simulink subsystem "Get_Lanes_and_Return_Map"  (R2022b)
settings: Solver=VariableStepAuto  StartTime=0.0  StopTime=10.0  RelTol=1e-3
settings Model: Creator=User  LastModifiedBy=User

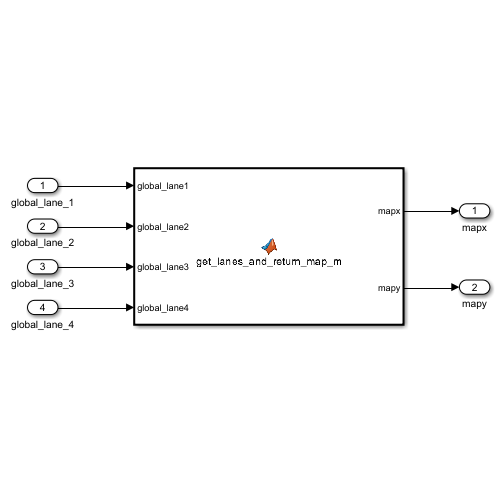
[thumbnail: Simulink's stored preview of the top-level diagram]
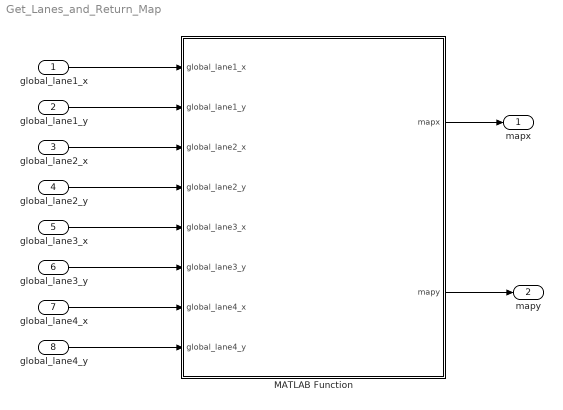
== system Get_Lanes_and_Return_Map ==
  global_lane1_x : Inport
  global_lane1_y : Inport  Port=2
  global_lane2_x : Inport  Port=3
  global_lane2_y : Inport  Port=4
  global_lane3_x : Inport  Port=5
  global_lane3_y : Inport  Port=6
  global_lane4_x : Inport  Port=7
  global_lane4_y : Inport  Port=8
  MATLAB Function : MATLAB Function  TreatAsAtomicUnit=on
  mapx : Outport
  mapy : Outport  Port=2
  wires:
  MATLAB Function/2(mapy) -> mapy/1
  MATLAB Function/1(mapx) -> mapx/1
  global_lane1_y/1 -> MATLAB Function/2(global_lane1_y)
  global_lane1_x/1 -> MATLAB Function/1(global_lane1_x)
  global_lane2_x/1 -> MATLAB Function/3(global_lane2_x)
  global_lane2_y/1 -> MATLAB Function/4(global_lane2_y)
  global_lane3_x/1 -> MATLAB Function/5(global_lane3_x)
  global_lane3_y/1 -> MATLAB Function/6(global_lane3_y)
  global_lane4_x/1 -> MATLAB Function/7(global_lane4_x)
  global_lane4_y/1 -> MATLAB Function/8(global_lane4_y)

== matlab function Get_Lanes_and_Return_Map/MATLAB Function ==
  data: global_lane1_x input; mapx output; global_lane1_y input; global_lane2_x input; global_lane2_y input; mapy output; global_lane3_x input; global_lane3_y input; global_lane4_x input; global_lane4_y input
function [mapx, mapy] = get_lanes_and_return_map_m(global_lane1_x, global_lane1_y, global_lane2_x, global_lane2_y, global_lane3_x, global_lane3_y, global_lane4_x, global_lane4_y)
    [mapx, mapy] = get_lanes_and_return_map(global_lane1_x, global_lane1_y, global_lane2_x, global_lane2_y, global_lane3_x, global_lane3_y, global_lane4_x, global_lane4_y);
    
end
